simulink model "DiagCCaller_TestHarness"  (R2019a)
settings: Solver=FixedStepDiscrete  StartTime=0.0  StopTime=10.0  FixedStep=0.1  RelTol=1e-3  EnableMultiTasking=on
undefined symbols (not defined in the file): Dem_EventStatusType, sigbuilder_block
(part 4 of 4)

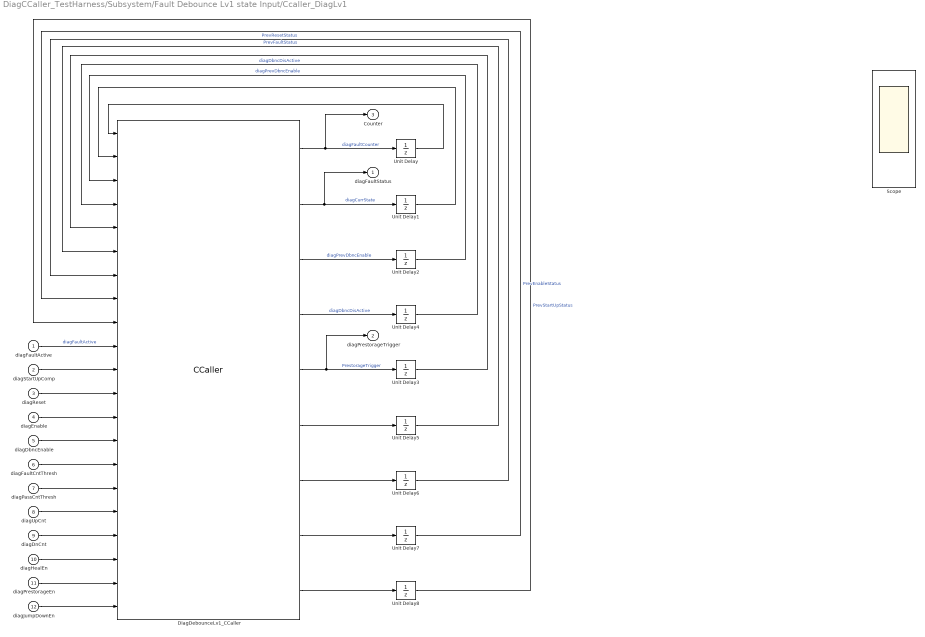
== system DiagCCaller_TestHarness/Subsystem/Fault Debounce Lv1 state Input/Ccaller_DiagLv1 ==
  diagFaultActive : Inport
  diagStartUpComp : Inport  Port=2
  diagReset : Inport  Port=3
  diagEnable : Inport  Port=4
  diagDbncEnable : Inport  Port=5
  diagFaultCntThresh : Inport  Port=6
  diagPassCntThresh : Inport  Port=7
  diagUpCnt : Inport  Port=8
  diagDnCnt : Inport  Port=9
  diagHealEn : Inport  Port=10
  diagPrestorageEn : Inport  Port=11
  diagJumpDownEn : Inport  Port=12
  DiagDebounceLv1_CCaller : CCaller  FunctionName=DiagDebounceLv1  PortSpecificationStruct="%)30     .    <\"$   8    (     @         %    \"    !4    !     0         %  0 \"0    $    V    07)G3F%M90  4&]R=$YA;64 4V-O<&4     26YD97@     5'EP90      4VEZ90         .    0     8    (    !          %    \"     $    0     0         0    $    &1I86=&875L=$-O=6YT97(.    0     8    (    !          %    \"     $    0     0         0    $    &1I86=&875L=$-O=6YT97(.    0     8    (    !          %  ...(+11158 chars)"
  Scope : Scope  NumInputPorts=8
  Unit Delay : UnitDelay  SampleTime=-1  HasFrameUpgradeWarning=on
      settings: AttributesFormatString=%<InitialCondition>
  Unit Delay1 : UnitDelay  InitialCondition=uint8(32)  SampleTime=-1  HasFrameUpgradeWarning=on
      settings: AttributesFormatString=%<InitialCondition>
  Unit Delay{2..8} (7 alike) : UnitDelay  InitialCondition=false  SampleTime=-1  HasFrameUpgradeWarning=on
      settings: AttributesFormatString=%<InitialCondition>
  diagFaultStatus : Outport
  diagPrestorageTrigger : Outport  Port=2
  Counter : Outport  Port=3  OutputWhenDisabled=reset  InitialOutput=Dem_EventStatusType.DEM_EVENT_STATUS_INIT
  wires:
  Unit Delay4/1 -> DiagDebounceLv1_CCaller/4  "diagDbncDisActive"
  DiagDebounceLv1_CCaller/4 -> Unit Delay4/1  "diagDbncDisActive"
  Unit Delay3/1 -> DiagDebounceLv1_CCaller/5
  DiagDebounceLv1_CCaller/5 -> Unit Delay3/1, diagPrestorageTrigger/1  "PrestorageTrigger"
  Unit Delay2/1 -> DiagDebounceLv1_CCaller/3  "diagPrevDbncEnable"
  DiagDebounceLv1_CCaller/3 -> Unit Delay2/1  "diagPrevDbncEnable"
  Unit Delay1/1 -> DiagDebounceLv1_CCaller/2
  DiagDebounceLv1_CCaller/2 -> Unit Delay1/1, diagFaultStatus/1  "diagCurrState"
  Unit Delay/1 -> DiagDebounceLv1_CCaller/1
  DiagDebounceLv1_CCaller/1 -> Counter/1, Unit Delay/1  "diagFaultCounter"
  DiagDebounceLv1_CCaller/6 -> Unit Delay5/1
  DiagDebounceLv1_CCaller/7 -> Unit Delay6/1
  DiagDebounceLv1_CCaller/8 -> Unit Delay7/1
  Unit Delay5/1 -> DiagDebounceLv1_CCaller/6  "PrevFaultStatus"
  Unit Delay6/1 -> DiagDebounceLv1_CCaller/7  "PrevResetStatus"
  Unit Delay7/1 -> DiagDebounceLv1_CCaller/8  "PrevEnableStatus"
  DiagDebounceLv1_CCaller/9 -> Unit Delay8/1
  diagJumpDownEn/1 -> DiagDebounceLv1_CCaller/21
  diagPrestorageEn/1 -> DiagDebounceLv1_CCaller/20
  diagHealEn/1 -> DiagDebounceLv1_CCaller/19
  diagDnCnt/1 -> DiagDebounceLv1_CCaller/18
  diagUpCnt/1 -> DiagDebounceLv1_CCaller/17
  diagPassCntThresh/1 -> DiagDebounceLv1_CCaller/16
  diagFaultCntThresh/1 -> DiagDebounceLv1_CCaller/15
  diagDbncEnable/1 -> DiagDebounceLv1_CCaller/14
  diagEnable/1 -> DiagDebounceLv1_CCaller/13
  diagReset/1 -> DiagDebounceLv1_CCaller/12
  diagStartUpComp/1 -> DiagDebounceLv1_CCaller/11
  diagFaultActive/1 -> DiagDebounceLv1_CCaller/10  "diagFaultActive"
  Unit Delay8/1 -> DiagDebounceLv1_CCaller/9  "PrevStartUpStatus"
